simulink model "nyquist_stab_mod"  (R2013a)
settings: Solver=ode45  StartTime=0.0  StopTime=10.0  RelTol=1e-3
values from neighbouring files (symbols this model uses):
  K = Kk(i)    [RT_wok_aufgabe.m]    (also in nyquist_stabil.m = 0.2; s_schrittantwort.m = 1; servo_4_proc.m = 1)
  Kp = 1    [RT_dennis_draussen.m]    (also in RT_reglersynthesePDF.m = 20; nyquist_stabil.m; regelungstechnik.m; reglersynthesePDFnoTuning.m = 20)
  T1 = 1    [nyquist_stabil.m]    (also in s_schrittantwort.m = 7)
settings Model: Creator=mainster  LastModifiedBy=mainster

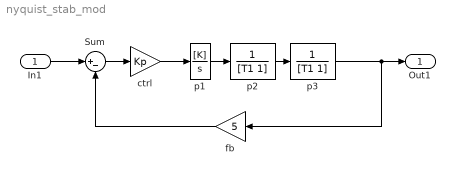
== system nyquist_stab_mod ==
  In1 : Inport
  Sum : Sum  Inputs=|+-
  ctrl : Gain  Gain=Kp
  fb : Gain  Gain=5
  p1 : TransferFcn  Numerator=[K]  Denominator=[1 0]
  p2 : TransferFcn  Denominator=[T1 1]
  p3 : TransferFcn  Denominator=[T1 1]
  Out1 : Outport
  wires:
  Sum/1 -> ctrl/1
  fb/1 -> Sum/2
  ctrl/1 -> p1/1
  p1/1 -> p2/1
  p2/1 -> p3/1
  p3/1 -> Out1/1, fb/1
  In1/1 -> Sum/1
